simulink model "NeuronalNetwork"  (R2019b)
settings: Solver=VariableStepAuto  StartTime=0.0  StopTime=10.0  RelTol=1e-3
libraries: neural x1006
(part 6 of 11)

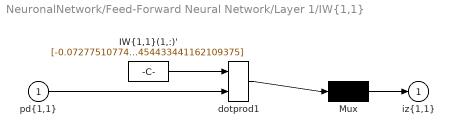
== system NeuronalNetwork/Feed-Forward Neural Network/Layer 1/IW{1,1} ==
  "pd{1,1}" : Inport  PortDimensions=1001  SampleTime=0.1
      mask Display: e = 0.06;c1 = [120 230 180]/255;c2 = ([120 230 180]+0)/(256+128);c3 = ([120 230 180]+128)/(256+128);patch([0 1 1 0],[0 0 1 1],c1);patch([0 1 1 1-e 1-e 0+e],[0 0 1 1-e 0+e 0+e],c2);patch([0 0 1 1-e 0+e 0+e],[0 1 1 1-e 1-e 0+e],c3);plot([0 1 1 0 0],[0 0 1 1 0]);
  "IW{1,1}(1,:)'" : Constant  Value=[-0.072775107747280909364917533821426331996917724609375;0.0394548788635098734989270496953395195305347442626953125;0.01012162685570140545354700378766210633330047130584716796875;0.0231203356415073495166989658855527522973716259002685546875;0.02020080557271976273714386707069934345781803131103515625;0.035131699392428668293764104646470514126121997833251953125;0.058069514355718353237900686281136586330831050872802734375;0.0248737271763740108720952548537752591073513031005859375;-0.05686994605112295764204333181623951531946659088134765625;0.0320440751475139784520962393798981793224811553955078125;-0.00791190741387180936083911575451566022820770740509033203125;0.021136625247377506531254454102963791228830814361572265625;0.022323089446683132275328631521915667690336704254150390625;0.026742736184336486637835861301937256939709186553955078125;-0.06614228432952172498371368192238151095807552337646484375;-0.041386005435294935528300896976361400447785854339599609375;-0.049777499487331421101909967319443239830434322357177734375;0.06424680322796551268371700871284701861441135406494140625;0.0022834896529049485136564356935195974074304103851318359375;0.025991335919095130690958939112533698789775371551513671875;0.0251572654682002648518501786156775779090821743011474609375;-0.062748938666416342879728063053335063159465789794921875;-0.0412180597263457626500127162216813303530216217041015625;-0.032355197043461021710886171831589308567345142364501953125;0.062033074557632579548727136398156289942562580108642578125;-0.04061415197016758626968879752894281409680843353271484375;-0.037687810552769519800708764023511321283876895904541015625;0.0264301987542764245386894828016011160798370838165283203125;0.022262300245454787195331647353668813593685626983642578125;0.0305360296531792078933431611176274600438773632049560546875;0.050539840898083020215292293642050935886800289154052734375;0.0340770600054231265207960177576751448214054107666015625;-0.07204827419684688150081086632781079970300197601318359375;0.01255559938764767673180511309283247101120650768280029296875;0.06309949805322685734143561830933322198688983917236328125;-0.0612172288370917971889184627798385918140411376953125;0.00817993988469976375521586220429526292718946933746337890625;0.0645876384448602625099056240287609398365020751953125;-0.045059189181758711739700373755113105289638042449951171875;0.0037960110759924924235531040750402098638005554676055908203125;-0.055960731551798557903421027504009543918073177337646484375;0.0372901657931143659663320022445986978709697723388671875;-0.0277855938520934313273880178485342185012996196746826171875;-0.046900076668728141182640456463559530675411224365234375;0.07202271457806264098877591095515526831150054931640625;0.031907875469494591247343606710273888893425464630126953125;0.048822719049413869363274187662682379595935344696044921875;0.027469031275259118973774974392654257826507091522216796875;0.0283958582902909088818699245848620194010436534881591796875;0.004629032860517649262954709143969012075103819370269775390625;-0.046648268889731558939359956639236770570278167724609375;-0.0010471125348824159191629679099833083455450832843780517578125;0.008926449452265276807150229387843864969909191131591796875;0.049217061038308453080336590801380225457251071929931640625;-0.0445470995639002664834293909734697081148624420166015625;0.004159821673042758856386758026246752706356346607208251953125;0.04614825909513353696667081749183125793933868408203125;-0.021723305715046083153030309631503769196569919586181640625;0.007159621411425333599443110443871773895807564258575439453125;0.03259913083009420564639668782547232694923877716064453125;-0.044600508758804037479084314554711454547941684722900390625;0.021552596024937954732880740493783378042280673980712890625;-0.07494860823653275161415621141713927499949932098388671875;0.001975544362883157635535358309653020114637911319732666015625;0.0104690385152326377593556827605425496585667133331298828125;-0.0739069843110099766736453830162645317614078521728515625 ...(+56224 chars)]
      mask Display: e = 0.06;c1 = [120 150 230]/255;c2 = ([120 150 230]+0)/383;c3 = ([120 150 230]+128)/383;patch([0 1 1 0],[0 0 1 1],c1);patch([0 1 1 1-e 1-e 0+e],[0 0 1 1-e 0+e 0+e],c2);patch([0 0 1 1-e 0+e 0+e],[0 1 1 1-e 1-e 0+e],c3);plot([0 1 1 0 0],[0 0 1 1 0]);disp('Weights');
  Mux : Mux  Inputs=1
      mask Display: e = 0.06;c1 = [120 150 230]/255;c2 = ([120 150 230]+0)/383;c3 = ([120 150 230]+128)/383;patch([0 1 1 0],[0 0 1 1],c1);patch([0 1 1 1-e 1-e 0+e],[0 0 1 1-e 0+e 0+e],c2);patch([0 0 1 1-e 0+e 0+e],[0 1 1 1-e 1-e 0+e],c3);plot([0 1 1 0 0],[0 0 1 1 0]);disp('Mux');
  dotprod1 : neural/Weight Functions/dotprod
      settings: SourceProductName=Deep Learning Toolbox
  "iz{1,1}" : Outport
      mask Display: e = 0.06;c1 = [120 230 180]/255;c2 = ([120 230 180]+0)/(256+128);c3 = ([120 230 180]+128)/(256+128);patch([0 1 1 0],[0 0 1 1],c1);patch([0 1 1 1-e 1-e 0+e],[0 0 1 1-e 0+e 0+e],c2);patch([0 0 1 1-e 0+e 0+e],[0 1 1 1-e 1-e 0+e],c3);plot([0 1 1 0 0],[0 0 1 1 0]);
  wires:
  "IW{1,1}(1,:)'"/1 -> dotprod1/1
  "pd{1,1}"/1 -> dotprod1/2
  dotprod1/1 -> Mux/1
  Mux/1 -> "iz{1,1}"/1
